simulink model "System"  (R2020a)
settings: Solver=VariableStepAuto  StartTime=0.0  StopTime=16.5  FixedStep=0.005  RelTol=1e-2
libraries: fmu_me_lib x1
settings Model: Creator=meagh

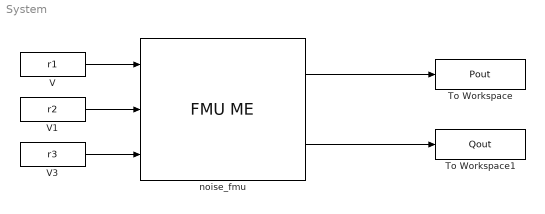
== system System ==
  To Workspace : ToWorkspace  VariableName=Pout  SaveFormat=Timeseries  SampleTime=-1
  To Workspace1 : ToWorkspace  VariableName=Qout  SaveFormat=Timeseries  SampleTime=-1
  V : FromWorkspace  VariableName=r1
  V1 : FromWorkspace  VariableName=r2
  V3 : FromWorkspace  VariableName=r3
  noise_fmu : fmu_me_lib/FMU ME  Description=Simulates an FMU for Model Exchange 1.0 or Model Exchange 2.0.  dummy=0
  wires:
  V/1 -> noise_fmu/1
  V1/1 -> noise_fmu/2
  noise_fmu/1 -> To Workspace/1
  V3/1 -> noise_fmu/3
  noise_fmu/2 -> To Workspace1/1
